simulink library "XXCopter_Control"  (R2015a)
settings: Solver=ode45  SolverMode=SingleTasking  StartTime=0.0  StopTime=10.0  RelTol=1e-3
undefined symbols (not defined in the file or in its folder): a, C_d0, h, h_FA, h_M, I_prop, I_tube, J_FA, J_T, m_FA, m_M, m_prop, Newton, omega_n, R, Raphson, rho, sigma, T_ctrl, theta_0, theta_1, Throtle_TTO_vec, TO_map_Omega, TO_map_Throtle, v_i0, v_i_adim, Vx_adim, Vz_adim, xi
undefined symbols (not defined in the file): direct_feedforward, l, l_arm, Rotation_sign, T_sim
libraries: vrlib x16, XXCopter_Control x10, aerolibutil x3, qcatlib x1, dspinverses x1
(part 2 of 2)

== system XXCopter_Control/Normalize 4D vector/4D vec norm/norm^2rm ==
  v : Inport
  Demux : Demux
  Product{,1..3} (4 alike) : Product
  Sum : Sum  Inputs=4
  norm(v) : Outport
  wires:
  Product3/1 -> Sum/4
  Demux/4 -> Product3/1, Product3/2
  Product2/1 -> Sum/3
  Demux/3 -> Product2/1, Product2/2
  v/1 -> Demux/1
  Sum/1 -> norm(v)/1
  Product/1 -> Sum/1
  Product1/1 -> Sum/2
  Demux/1 -> Product/1, Product/2
  Demux/2 -> Product1/1, Product1/2

== matlab function XXCopter_Control/Gyroscopic Moments  to C/Arm Inertia1 ==
  data: T_FAFb input; Arm_axis input; J_Arm output; I_tube parameter; I_prop parameter; h_FA parameter; h_M parameter; m_FA parameter; m_M parameter; m_prop parameter; h parameter
function J_Arm  = Arm_inertia(T_FAFb,Arm_axis, I_tube, I_prop, h_FA, h_M, m_FA, m_M, m_prop, h)


r_FAO=Arm_axis+T_FAFb*[0;0;-h_FA];
r_MO=Arm_axis+T_FAFb*[0;0;-h_M];
r_po=Arm_axis+T_FAFb*[0;0;-h];

I_FA = m_FA*[ r_FAO(2)^2+r_FAO(3)^2,r_FAO(1)*r_FAO(2),r_FAO(1)*r_FAO(3);...
            r_FAO(1)*r_FAO(2), r_FAO(1)^2+r_FAO(3)^2, r_FAO(2)*r_FAO(3);...
            r_FAO(1)*r_FAO(3),r_FAO(2)*r_FAO(3), r_FAO(1)^2+r_FAO(2)^2];
I_M = m_M*[ r_MO(2)^2+r_MO(3)^2,r_MO(1)*r_MO(2),r_MO(1)*r_MO(3);...
            r_MO(1)*r_MO(2), r_MO(1)^2+r_MO(3)^2, r_MO(2)*r_MO(3);...
            r_MO(1)*r_MO(3),r_MO(2)*r_MO(3), r_MO(1)^2+r_MO(2)^2];
I_steiner = m_prop*[ r_po(2)^2+r_po(3)^2,r_po(1)*r_po(2),r_po(1)*r_po(3);...
            r_po(1)*r_po(2), r_po(1)^2+r_po(3)^2, r_po(2)*r_po(3);...
            r_po(1)*r_po(3),r_po(2)*r_po(3), r_po(1)^2+r_po(2)^2];

% J_Arm = T_FAFb*I_prop*T_FAFb'+ I_tube +I_FA+I_M+I_steiner;
J_Arm = T_FAFb*I_prop*T_FAFb' +I_FA+I_M+I_steiner; % Quitamos el tubo ya que es insignificante y hay que calcularlo para cada brazo

== matlab function XXCopter_Control/Arm Dynamics  to C/Aerodynamics Propeller/Prop Coefficients to C ==
  data: lambda input; C_T output; mu input; C_H output; C_MH output; C_Q output; sigma parameter; C_d0 parameter; a parameter; theta_0 parameter; theta_1 parameter
function [C_T,C_H,C_MH,C_Q] = Aero_coeff(lambda,mu, sigma, C_d0, a, theta_0, theta_1)


C_T = sigma*a/4*(theta_0*(2/3+mu^2) +theta_1/2*(1+mu^2) -  lambda );
C_Q =    +sigma*a/4*( 2/3*theta_0 - lambda + theta_1/2)*lambda + sigma*C_d0/8*(1+mu^2);   % Always positive!!!


C_H = sigma*a/4*mu*lambda*(theta_0+theta_1/2) + sigma*C_d0/4*mu; 
C_MH= sigma*a/4*( 2/3*theta_0*mu-1/2*lambda*mu+theta_1*mu/2  );

== matlab function XXCopter_Control/Servos Dynamics  to C/Compute rise time ==
  data: xi input; omega_n input; t_r output
function t_r = rise_time(xi,omega_n)
t_r = 2.2/omega_n;
if xi<1
    t_r = (2.16*xi+0.6)/omega_n;
elseif xi>=1
    t_r = 2.2/omega_n;
end

== matlab function XXCopter_Control/Gravity Force and Moment ==
  data: q input; F_g_b output; M_g_b output; mass input; CG input; g parameter
function [F_g_b,M_g_b]   = Grav_Forces_and_Mom( q,mass,CG, g)

Prod=HamiltonProduct([q(1);-q(2);-q(3);-q(4)],HamiltonProduct([0;0;0;mass*g],[q(1);q(2);q(3);q(4)]) ); % q* . g .q

F_g_b= Prod(2:4);
M_g_b=cross(CG,F_g_b);


function Product= HamiltonProduct( a,b )

Product=[ a(1)*b(1)-a(2)*b(2)-a(3)*b(3)-a(4)*b(4) ; a(1)*b(2)+a(2)*b(1)+a(3)*b(4)-a(4)*b(3)  ; a(1)*b(3)-a(2)*b(4)+a(3)*b(1)+a(4)*b(2)  ; a(1)*b(4)+a(2)*b(3)-a(3)*b(2)+a(4)*b(1) ];

== matlab function XXCopter_Control/Control allocator 4 coder/Embedded MATLAB Function ==
  data: v input; u output size=[9,1]; u_ant input; W input; ud input; B input; plim input; rlim input; T input size=1; Wv input; Wu input; gammma input size=1; imax input; W_out output size=[9,1]
function [u , W_out ] = qp_ca_WLS(v,u_ant,W,ud,B,plim,rlim,T,Wv,Wu, gammma,imax)


% Formulate as a regular QP problem: min ||Wu(u-ud)||

% Overall position limits
if isempty(rlim)
    umin = plim(:,1);
    umax = plim(:,2);
else
    umin = max(plim(:,1),u_ant+rlim(:,1)*T);
    umax = min(plim(:,2),u_ant+rlim(:,2)*T);
end

% Start with the last
u=u_ant;
W_out=W;

% Number of variables
m = length(umin);
%   Wu*(u-ud)
% Set default values of optional arguments
if nargin < 11
    imax = 100; % Heuristic value
    [k,m] = size(B);
    if nargin < 10, u = (umin+umax)/2; W = zeros(m,1); end
    if nargin < 8,  gammma = 1e6;       end
    if nargin < 7,  ud = zeros(m,1); end
    if nargin < 6,  Wu = eye(m);     end
    if nargin < 5,  Wv = eye(k);     end
end

gammma_sq = sqrt(gammma);
A = [gammma_sq*Wv*B ; Wu];
b = [gammma_sq*Wv*v ; Wu*ud];

% Initial residual.
d = b - A*u;
% Determine indeces of free variables.
i_free = zeros(size(W));
i_free = (W==0);

% Iterate until optimum is found or maximum number of iterations
% is reached.
for iter = 1:imax
    % ----------------------------------------
    %  Compute optimal perturbation vector p.
    % ----------------------------------------
    
    % Eliminate saturated variables.
    A_free = A(:,i_free);
    % Solve the reduced optimization problem for free variables.
    p_free = A_free\d;
    % Zero all perturbations corresponding to active constraints.
    p = zeros(m,1);
    % Insert perturbations from p_free into free the variables.
    p(i_free) = p_free;
    
    % ----------------------------
    %  Is the new point feasible?
    % ----------------------------
    
    u_opt = u + p;
    infeasible = (u_opt < umin) | (u_opt > umax);
    
    if ~any(infeasible(i_free))
        
        % ----------------------------
        %  Yes, check for optimality.
        % ----------------------------
        
        % Update point and residual.
        u = u_opt;
        d = d - A_free*p_free;
        % Compute Lagrangian multipliers.
        lambda = W.*(A'*d);
        % Are all lambda non-negative?
        if min(lambda) >= -eps
            % / ------------------------ \
            % | Optimum found, bail out. |
            % \ ------------------------ /
            return;
        end
        
        % --------------------------------------------------
        %  Optimum not found, remove one active constraint.
        % --------------------------------------------------
        
        % Remove constraint with most negative lambda from the
        % working set.
        [lambda_neg,i_neg] = min(lambda);
        W_out(i_neg) = 0;
        i_free(i_neg) = 1;
        
    else
        
        % ---------------------------------------
        %  No, find primary bounding constraint.
        % ---------------------------------------
        
        % Compute distances to the different boundaries. Since alpha < 1
        % is the maximum step length, initiate with ones.
        dist = ones(m,1);
        i_min = i_free & p<0;
        i_max = i_free & p>0;
        
        dist(i_min) = (umin(i_min) - u(i_min)) ./ p(i_min);
        dist(i_max) = (umax(i_max) - u(i_max)) ./ p(i_max);
        
        % Proportion of p to travel
        [alpha,i_alpha] = min(dist);
        % Update point and residual.
        u = u + alpha*p;
        d = d - A_free*alpha*p_free;
        
        % Add corresponding constraint to working set.
        W_out(i_alpha) = sign(p(i_alpha));
        i_free(i_alpha) = 0;
        
    end
    
    
end


end

== matlab function XXCopter_Control/Arms Kinematics  to C/DCM Arm ==
  data: arm_no input; eta input; T_Fb_FA output; gamma input
function T_Fb_FA = DCM_Arm(arm_no,eta, gamma)
if arm_no==1
    T_Fb_FA = [ cos(gamma), sin(eta)*sin(gamma), -cos(eta)*sin(gamma);...
            0,cos(eta),sin(eta);...
            sin(gamma),-cos(gamma)*sin(eta),cos(gamma)*cos(eta) ];
elseif arm_no==2 || arm_no==3
    T_Fb_FA = [cos(eta),0,-sin(eta) ;...
            sin(eta)*sin(gamma),cos(gamma),cos(eta)*sin(gamma);...
            sin(eta)*cos(gamma),-sin(gamma),cos(eta)*cos(gamma)];
else
    error('That is not right: Chose a right arm'); 
end

== matlab function XXCopter_Control/Prop Coefficients to C ==
  data: lambda input; C_T output; mu input; C_H output; C_MH output; C_Q output; sigma parameter; C_d0 parameter; a parameter; theta_0 parameter; theta_1 parameter
function [C_T,C_H,C_MH,C_Q] = Aero_coeff(lambda,mu, sigma, C_d0, a, theta_0, theta_1)


C_T = sigma*a/4*(theta_0*(2/3+mu^2) +theta_1/2*(1+mu^2) -  lambda );
C_Q =    +sigma*a/4*( 2/3*theta_0 - lambda + theta_1/2)*lambda + sigma*C_d0/8*(1+mu^2);   % Always positive!!!


C_H = sigma*a/4*mu*lambda*(theta_0+theta_1/2) + sigma*C_d0/4*mu; 
C_MH= sigma*a/4*( 2/3*theta_0*mu-1/2*lambda*mu+theta_1*mu/2  );
